simulink model "Parameter_estimation_using_simulink"  (R2016a)
settings: Solver=ode4  StartTime=0.0  StopTime=10.0  FixedStep=0.01  RelTol=1e-3
undefined symbols (not defined in the file or in its folder): c_a, CL_0, CL_alpha, CL_alpha_dot, CL_dele, param_states
settings Model: Creator=PD Banneheka  LastModifiedBy=PD Banneheka
settings GRTTargetCC: GeneratePreprocessorConditionals=Use local settings

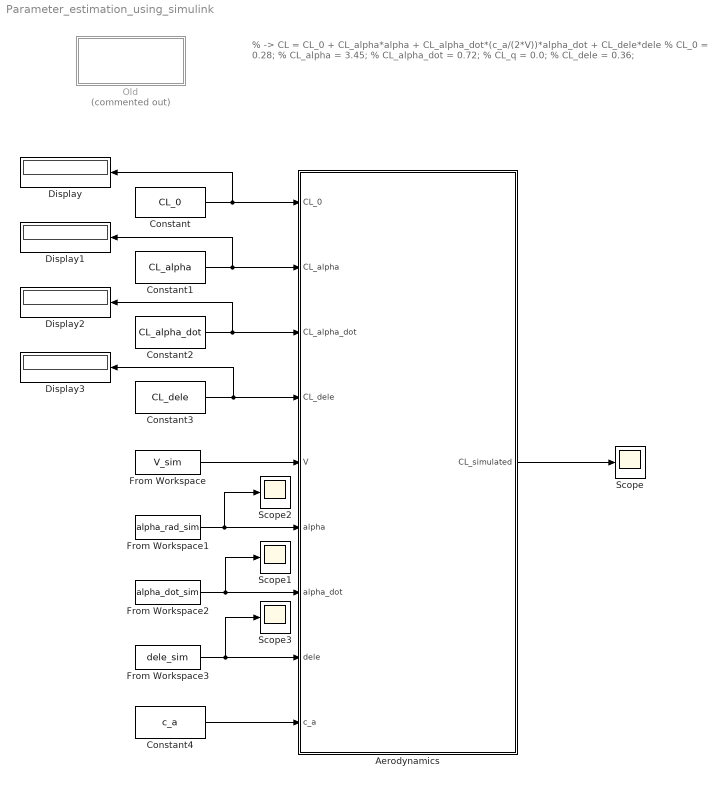
== system Parameter_estimation_using_simulink ==
  note: % -> CL = CL_0 + CL_alpha*alpha + CL_alpha_dot*(c_a/(2*V))*alpha_dot + CL_dele*dele
      | % CL_0             = 0.28;
      | % CL_alpha        = 3.45;
      | % CL_alpha_dot    = 0.72;
      | % CL_q            = 0.0;
      | % CL_dele         = 0.36;
  Aerodynamics : MATLAB Function  TreatAsAtomicUnit=on
  Constant : Constant  Value=CL_0
  Constant1 : Constant  Value=CL_alpha
  Constant2 : Constant  Value=CL_alpha_dot
  Constant3 : Constant  Value=CL_dele
  Constant4 : Constant  Value=c_a
  Display{,1..3} (4 alike) : Display
  From Workspace : FromWorkspace  VariableName=V_sim  SampleTime=0
  From Workspace1 : FromWorkspace  VariableName=alpha_rad_sim  SampleTime=0
  From Workspace2 : FromWorkspace  VariableName=alpha_dot_sim  SampleTime=0
  From Workspace3 : FromWorkspace  VariableName=dele_sim  SampleTime=0
  Old : Subsystem  Commented=on
  Scope{,1..3} (4 alike) : Scope
  wires:
  Constant1/1 -> Display1/1, Aerodynamics/2(CL_alpha)
  Constant2/1 -> Display2/1, Aerodynamics/3(CL_alpha_dot)
  Constant3/1 -> Display3/1, Aerodynamics/4(CL_dele)
  From Workspace/1 -> Aerodynamics/5(V)
  From Workspace1/1 -> Aerodynamics/6(alpha), Scope2/1
  From Workspace2/1 -> Aerodynamics/7(alpha_dot), Scope1/1
  From Workspace3/1 -> Scope3/1, Aerodynamics/8(dele)
  Aerodynamics/1(CL_simulated) -> Scope/1
  Constant4/1 -> Aerodynamics/9(c_a)
  Constant/1 -> Display/1, Aerodynamics/1(CL_0)

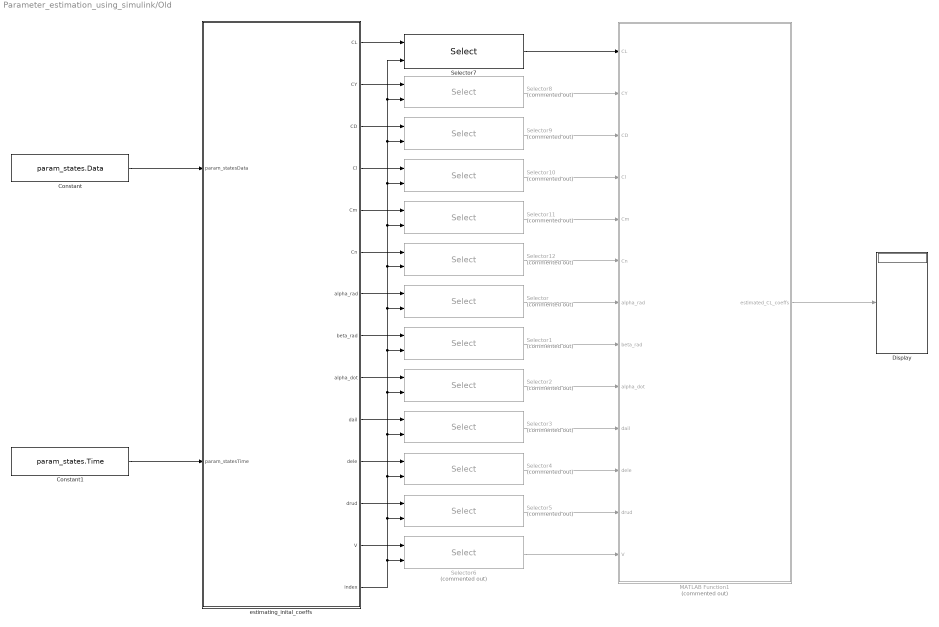
== system Parameter_estimation_using_simulink/Old ==
  Constant : Constant  Value=param_states.Data  VectorParams1D=off
  Constant1 : Constant  Value=param_states.Time  VectorParams1D=off
  Display : Display
  MATLAB Function1 : MATLAB Function  Commented=on  TreatAsAtomicUnit=on
  Selector{,1..6,8..12} (12 alike) : Selector  Commented=on  InputPortWidth=3  IndexOptions=Index vector (port)  Indices=[1 3]  OutputSizes=1
  Selector7 : Selector  IndexOptions=Index vector (port)  Indices=[1:3]  OutputSizes=1
  estimating_inital_coeffs : MATLAB Function  TreatAsAtomicUnit=on
  wires:
  estimating_inital_coeffs/7(alpha_rad) -> Selector/1
  estimating_inital_coeffs/11(dele) -> Selector4/1
  Constant1/1 -> estimating_inital_coeffs/2(param_statesTime)
  estimating_inital_coeffs/9(alpha_dot) -> Selector2/1
  estimating_inital_coeffs/8(beta_rad) -> Selector1/1
  Constant/1 -> estimating_inital_coeffs/1(param_statesData)
  MATLAB Function1/1(estimated_CL_coeffs) -> Display/1
  estimating_inital_coeffs/10(dail) -> Selector3/1
  Selector5/1 -> MATLAB Function1/12(drud)
  Selector9/1 -> MATLAB Function1/3(CD)
  estimating_inital_coeffs/2(CY) -> Selector8/1
  Selector2/1 -> MATLAB Function1/9(alpha_dot)
  Selector11/1 -> MATLAB Function1/5(Cm)
  Selector8/1 -> MATLAB Function1/2(CY)
  estimating_inital_coeffs/13(V) -> Selector6/1
  Selector7/1 -> MATLAB Function1/1(CL)
  estimating_inital_coeffs/5(Cm) -> Selector11/1
  Selector1/1 -> MATLAB Function1/8(beta_rad)
  Selector3/1 -> MATLAB Function1/10(dail)
  estimating_inital_coeffs/1(CL) -> Selector7/1
  Selector6/1 -> MATLAB Function1/13(V)
  Selector12/1 -> MATLAB Function1/6(Cn)
  estimating_inital_coeffs/12(drud) -> Selector5/1
  estimating_inital_coeffs/4(Cl) -> Selector10/1
  estimating_inital_coeffs/6(Cn) -> Selector12/1
  Selector4/1 -> MATLAB Function1/11(dele)
  estimating_inital_coeffs/14(index) -> Selector/2, Selector12/2, Selector11/2, Selector10/2, Selector9/2, Selector8/2, Selector7/2, Selector1/2, Selector2/2, Selector3/2, Selector4/2, Selector5/2, Selector6/2
  Selector10/1 -> MATLAB Function1/4(Cl)
  estimating_inital_coeffs/3(CD) -> Selector9/1
  Selector/1 -> MATLAB Function1/7(alpha_rad)

== matlab function Parameter_estimation_using_simulink/Old/estimating_inital_coeffs ==
  data: CL output; CY output; CD output; Cl output; Cm output; Cn output; alpha_rad output; beta_rad output; alpha_dot output; dail output; dele output; drud output; V output; index output size=100000; param_statesData input; param_statesTime input
function [CL,CY,CD,Cl,Cm,Cn,alpha_rad,beta_rad,alpha_dot,dail,dele,drud,V,index]= estimating_initial_coeffs(param_statesData,param_statesTime)

%param_file_list = dir('*param_states.mat');

%i = 3; % For file: '03_short_period_phugoid_spherical_constrained_0_8_param_states'
%filename = param_file_list(i).name;
%load(filename);

filename = '03_short_period_phugoid_spherical_constrained_0_8_param_states';

loads = zeros(size(param_statesData,1),19); % 19 is the length of the output of function 'estimated_loads'.

for ii = 1:size(param_statesData,1)
    loads(ii,:) = estimated_loads(param_statesData(ii,:)');
end

time = param_statesTime;

L_estimated = loads(:,1); % (N) (wind axes)
D_estimated = loads(:,2); % (N) (wind axes)
Y_estimated = loads(:,3); % (N) (wind axes)
l_estimated = loads(:,4); % (N.m) (body axes)
m_estimated = loads(:,5); % (N.m) (body axes)
n_estimated = loads(:,6); % (N.m) (body axes)
dail = loads(:,7); % Aileron (rad)
dele = loads(:,8); % Elevator (rad)
drud = loads(:,9); % Rudder (rad)

b_a = loads(end,10); % Wing span (m)f
c_a = loads(end,11); % Reference cord, MAC (m)
S_a = loads(end,12); % Wing area (m^2)
rho = loads(end,13); % Density (kg/m^3)];

V = loads(:,14); % Aircraft total speed (m/s)
p = loads(:,15); % (rad/sec) (body axes)
q = loads(:,16); % (rad/sec) (body axes)
r = loads(:,17); % (rad/sec) (body axes)

alpha_rad = loads(:,18); % (rad)
beta_rad = loads(:,19); % (rad)
deltaT = param_statesTime(2)-param_statesTime(1); % Time step (s)
alpha_dot_temp = diff(alpha_rad)/deltaT; % (rad/s)
%alpha_dot(end+1) = alpha_dot(end); % So that matrix dimensions are consistent
alpha_dot= [alpha_dot_temp; alpha_dot_temp(end)]; % So that matrix dimensions are consistent

% Total coefficients
CL = L_estimated./(0.5*rho*V.^2*S_a);
CD = D_estimated./(0.5*rho*V.^2*S_a);
CY = Y_estimated./(0.5*rho*V.^2*S_a);
Cl = l_estimated./(0.5*rho*V.^2*S_a*b_a);
Cm = m_estimated./(0.5*rho*V.^2*S_a*c_a);
Cn = n_estimated./(0.5*rho*V.^2*S_a*b_a);

[ time_period, startIdx, endIdx, index ] = analysis_time_for_simulink(filename,time);
%disp('Analysis start and end times:');
%disp(time_period, startIdx, endIdx);
%coder.extrinsic('find');
% startIdx = find(time==time_period(1));
% endIdx = find(time==time_period(2));

%index = [startIdx:endIdx];
%index = [startIdx:endIdx];
%index = [2000:4001];

== matlab function Parameter_estimation_using_simulink/Aerodynamics ==
  data: CL_0 input; CL_simulated output; CL_alpha input; CL_alpha_dot input; CL_dele input; V input; alpha input; alpha_dot input; dele input; c_a input
function CL_simulated = fcn(CL_0, CL_alpha, CL_alpha_dot, CL_dele, V, alpha, alpha_dot, dele, c_a)

CL_simulated = CL_0 + CL_alpha*alpha + CL_alpha_dot*(c_a/(2*V))*alpha_dot + CL_dele*dele;

== matlab function Parameter_estimation_using_simulink/Old/MATLAB Function1 ==
  data: CL input; CY input; CD input; Cl input; Cm input; Cn input; alpha_rad input; beta_rad input; alpha_dot input; dail input; dele input; drud input; estimated_CL_coeffs output; V input
function estimated_CL_coeffs = fcn(CL,CY,CD,Cl,Cm,Cn,alpha_rad,beta_rad,alpha_dot,dail,dele,drud,V)

% -> CL = CL_0 + CL_alpha*alpha + CL_alpha_dot*(c_a/(2*V))*alpha_dot + CL_dele*dele
% CL0             = 0.28;
% CL_alpha        = 3.45;
% CL_alpha_dot    = 0.72;
% CL_q            = 0.0;
% CL_dele         = 0.36;

% Using equation error method to estimate coefficients
X_CL = [ ones(length(alpha_rad),1) alpha_rad c_a./(2.*V).*alpha_dot dele];
estimated_CL_coeffs = ((X_CL'*X_CL)\X_CL')*CL;
